simulink model "MotMappedP1"  (R2020a)
settings: Solver=VariableStepAuto  StartTime=0.0  StopTime=inf  RelTol=1e-3  EnableMultiTasking=on
model workspace (MAT data in the model file):
  T_eff_bp = [0 20 40 60 80 100 120 140 160 180 200]
  T_t = [200 200 200 200 190.9859317 143.2394488 114.591559 95.49296586 81.85111359 71.61972439 63.66197724 57.29577951 52.08707228 47.74648293]
  Tc = 0.02
  efficiency_table = [52  78  80  82  82  80  78  78  76  74  70; 52  78  80  82  82  80  78  78  76  74  70; 52  78  84  86  86  86  86  84  84  82  82; 52  80  86  86  88  88  88  86  86  84  84; 52  80  86  88  88  88  88  88  86  86  86; 52  80  86  88  90  90  90  90  88  88  88; 52  82  88  90  91  91  92  92  92  91  91; 52  82  88  91  91  92  93  93  93  93  93; 52  84  90  92  92  93  93  93  93  93  93; 62  86  91  93  93  93  93  93  93  93  93; 66  86  91  93  93  93  93  93  93  93  93; 70  86  92  93  93  93  93  93  93  93  93; 70  86  92  93  93  93  93  93  93  93  93; 72  86  91  93  93  93  93  93  93  93  93]
  power_max = 30000
  torque_max = 200
  w_eff_bp = [0 500 1000 1432.391138 1500 2000 2500 3000 3500 4000 4500 5000 5500 6000]
libraries: autolibmappedmotor x1
settings Model: ModifiedByFormat=The MathWorks, Inc.  PauseTimes=10  Creator=The MathWorks, Inc.  LastModifiedBy=The MathWorks, Inc.
settings SolverCC: AutoInsertRateTranBlk=on  DecoupledContinuousIntegration=on
settings DataIOCC: DSMLogging=off  ReturnWorkspaceOutputs=off
settings DebuggingCC: ArithmeticOperatorsInVariantConditions=warning
settings ModelReferenceCC: PropagateSignalLabelsOutOfModel=off
settings SFSimCC: SimUseLocalCustomCode=off  CustomCodeUndefinedFunction=UseInterfaceOnly
settings RTWCC: RTWUseLocalCustomCode=off
settings CodeAppCC: StateflowObjectComments=on
settings GRTTargetCC: TargetLangStandard=C89/C90 (ANSI)
settings ConfigComp: CovMetricSettings=dsw  CovHtmlReporting=on  CovSaveCumulativeToWorkspaceVar=on  CovSaveSingleToWorkspaceVar=on  CovShowResultsExplorer=off  CovExternalEMLEnable=off
settings SimscapeCC: SimscapeNormalizeSystem=off

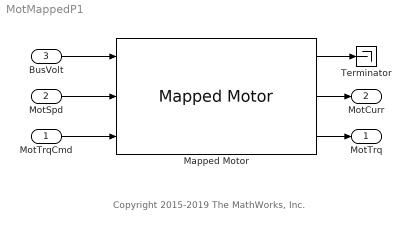
== system MotMappedP1 ==
  note: Copyright 2015-2019 The MathWorks, Inc.
  MotTrqCmd : Inport
  MotSpd : Inport  Port=2
  BusVolt : Inport  Port=3
  Mapped Motor : autolibmappedmotor/Mapped Motor  port_config=Speed  param_by=Tabulated torque-speed envelope  w_t=w_eff_bp.*pi/30  T_t=T_t  torque_max=torque_max  power_max=power_max  Tc=Tc  param_loss=Tabulated efficiency data  eff=100  w_eff=375  T_eff=0.08  Piron=0  Pbase=0  w_eff_bp=w_eff_bp.*pi/30  T_eff_bp=T_eff_bp  Temp_eff_bp=[233.15 293.15 373.15]  losses_table=[1 2;3 4]  losses_table_3d=cat(3,1.05*[1.49 1.67 2.21 3.10; 0.42 0.69 1.14 2.03; 0.06 0.24 0.78 1.68; 0.42 0.69 1.14 2.03; 1.49 1.67 2.21 3.10],[1.49 1.67 2.21 3.10; 0.42 0.69 1.14 2.03; 0.06 0.24 0.78 1.68; 0.42 0.69 1.14 2.03; 1.49 1.67 2.21 3.10],1.03*[1.49 1.67 2.21 3.10; 0.42 0.69 1.14 2.03; 0.06 0.24 0.78 1.68; 0.42 0.69 1.14 2.03; 1.49 1.67 2.21 3.10])  efficiency_table=efficiency_table  efficiency_table_3d=cat(3,90*ones(5,4),95*ones(5,4),92*ones(5,4))  J=5e-6  b=1e-5  omega_o=0  T_t_extended=[47.74648293 52.08707228 57.29577951 63.66197724 71.61972439 81.85111359 95.49296586 114.591559 143.2394488 190.9859317 200 200 200 200 200 200 200 190.9859317 143.2394488 114.591559 95.49296586 81.85111359 71.61972439 63.66197724 57.29577951 52.08707228 47.74648293]  w_t_extended=[-628.318530717959 -575.958653158129 -523.598775598299 -471.238898038469 -418.879020478639 -366.519142918809 -314.159265358979 -261.799387799149 -209.43951023932 -157.07963267949 -149.999649206931 -104.71975511966 -52.3598775598299 0 52.3598775598299 104.71975511966 149.999649206931 157.07963267949 209.43951023932 261.799387799149 314.159265358979 366.519142918809 418.879020478639 471.238898038469 523.598775598299 575.958653158129 628.318530717959]  KLossIron=0  KLossCopper=0  x_w_eff_vec=[-628.318530717959 -575.958653158129 -523.598775598299 -471.238898038469 -418.879020478639 -366.519142918809 -314.159265358979 -261.799387799149 -209.43951023932 -157.07963267949 -149.999649206931 -104.71975511966 -52.3598775598299 0 52.3598775598299 104.71975511966 149.999649206931 157.07963267949 209.43951023932 261.799387799149 314.159265358979 366.519142918809 418.879020478639 471.238898038469 523.598775598299 575.958653158129 628.318530717959]  x_T_eff_vec=[-200 -180 -160 -140 -120 -100 -80 -60 -40 -20 0 20 40 60 80 100 120 140 160 180 200]  x_tmp_eff_vec=[233.15 293.15 373.15]  x_losses_mat=[9458.558526937 8512.7026742433 7566.8468215496 6620.9909688559 5675.1351161622 4729.2792634685 3783.4234107748 2837.5675580811 2485.6557259172 2045.68823954684 0 1759.29188601028 2261.94671058465 2638.93782901542 3518.58377202057 4398.22971502571 5277.87565803085 6157.52160103599 7037.16754404113 7916.81348704627 8796.45943005141;8670.34531635892 7803.31078472303 6936.27625308713 6069.24172145124 5202.20718981535 4335.17265817946 3468.13812654357 2601.10359490768 2003.3344457674 1875.21421958461 0 1612.68422884276 1843.06769010601 2419.02634326414 3225.36845768552 4031.7105721069 4838.05268652828 5644.39480094966 6450.73691537104 7257.07902979242 8063.4211442138;7882.13210578084 7093.91889520275 6305.70568462467 5517.49247404659 4729.2792634685 3941.06605289042 3152.85284231233 2364.63963173425 1821.21313251582 1704.74019962237 0 1466.07657167524 1675.51608191456 2199.11485751285 2932.15314335047 3665.19142918809 4398.22971502571 5131.26800086333 5864.30628670094 6597.34457253856 7330.38285837618;7093.91889520275 6384.52700568248 5675.1351161622 4965.74322664193 4256.35133712165 3546.95944760138 2837.5675580811 2128.17566856083 1864.2417944379 1534.26617966013 0 1319.46891450771 1696.46003293849 1979.20337176157 2638.93782901542 3298.67228626928 3958.40674352314 4618.14120077699 5277.87565803085 5937.61011528471 6597.34457253856;6305.70568462467 5675.1351161622 5044.56454769974 4413.99397923727 3783.4234107748 3152.85284231233 2522.28227384987 1891.7117053874 1657.10381727813 1363.7921596979 0 1172.86125734019 1507.9644737231 1759.29188601028 2345.72251468038 2932.15314335047 3518.58377202057 4105.01440069066 4691.44502936075 5277.87565803085 5864.30628670094;5517.49247404658 4965.74322664193 4413.99397923727 3862.24473183261 3310.49548442795 2758.74623702329 2549.69838552215 1912.27378914161 1628.97396852804 1396.26340159546 0 1172.86125734019 1466.07657167524 1759.29188601028 2345.72251468038 2565.63400043166 3078.76080051799 3591.88760060433 4105.01440069066 4618.14120077699 5131.26800086332;4729.2792634685 4256.35133712165 3783.4234107748 3310.49548442795 2837.5675580811 2731.81969877373 2485.6557259172 1864.2417944379 1713.59599286716 1379.23579913698 0 1130.97335529233 1507.9644737231 1696.46003293849 2261.94671058465 2513.27412287183 2638.93782901542 3078.760800518 3518.58377202057 3958.40674352314 4398.22971502571;5178.44942899416 4660.60448609474 3642.42626503164 3187.12298190269 2731.81969877373 2589.22471449708 2071.37977159766 1745.32925199433 1427.99666072263 1149.36316594749 0 942.477796076938 1256.63706143592 1570.7963267949 1884.95559215388 2356.19449019234 2513.27412287183 2932.15314335047 3351.03216382911 4241.15008234622 4712.38898038469;5711.98664289054 5140.78797860148 4569.58931431243 3257.94793705608 2792.52680319093 2327.10566932577 1861.68453546062 1713.59599286716 1363.7921596979 1047.1975511966 0 837.758040957278 1172.86125734019 1507.9644737231 1675.51608191456 2094.39510239319 2513.27412287183 2932.15314335047 4021.23859659494 4523.8934211693 5026.54824574367;5114.22059886711 4602.7985389804 4091.37647909369 2998.79298751753 2570.39398930074 2141.99499108395 1713.59599286716 1285.19699465037 1022.84411977342 785.398163397448 0 628.318530717959 879.645943005142 1130.97335529233 1507.9644737231 1884.95559215388 2261.94671058465 2638.93782901543 3518.58377202057 3958.40674352314 4398.22971502571;5714.27235074022 5142.8451156662 3906.96760725029 3418.596656344 2454.53971429523 2045.44976191269 1636.35980953016 1465.11285271886 976.741901812573 749.998246034654 0 599.998596827723 839.998035558812 1259.99705333822 1439.99663238654 1799.99579048317 2159.9949485798 2939.99312445584 3359.99214223525 4319.98989715961 4799.98877462179;4597.45266378994 4137.70739741095 3191.45920364677 2792.52680319093 2045.68823954684 1704.74019962237 1363.7921596979 1022.84411977342 797.864800911693 590.726823751927 0 460.766922526503 670.206432765823 879.645943005142 1172.86125734019 1466.07657167524 1759.29188601028 ...(+4852 chars)]  x_losses_mat_3d=cat(3,[3.255 2.3205 1.7535 1.5645 1.7535 2.3205 3.255;2.1315 1.197 0.7245 0.441 0.7245 1.197 2.1315;1.764 0.819 0.252 0.063 0.252 0.819 1.764;2.1315 1.197 0.7245 0.441 0.7245 1.197 2.1315;3.255 2.3205 1.7535 1.5645 1.7535 2.3205 3.255],[3.1 2.21 1.67 1.49 1.67 2.21 3.1;2.03 1.14 0.69 0.42 0.69 1.14 2.03;1.68 0.78 0.24 0.06 0.24 0.78 1.68;2.03 1.14 0.69 0.42 0.69 1.14 2.03;3.1 2.21 1.67 1.49 1.67 2.21 3.1],[3.193 2.2763 1.7201 1.5347 1.7201 2.2763 3.193;2.0909 1.1742 0.7107 0.4326 0.7107 1.1742 2.0909;1.7304 0.8034 0.2472 0.0618 0.2472 0.8034 1.7304;2.0909 1.1742 0.7107 0.4326 0.7107 1.1742 2.0909;3.193 2.2763 1.7201 1.5347 1.7201 2.2763 3.193])  CalLossMapData={}  CalLossWithTempMapData={}  aMode=aMode  RefBlkName='autolibmappedmotor/Mapped Motor'
      settings: SourceProductBaseCode=PW,MT,VE,VP
  Terminator : Terminator
  MotTrq : Outport  VectorParamsAs1DForOutWhenUnconnected=off
  MotCurr : Outport  Port=2  VectorParamsAs1DForOutWhenUnconnected=off
  wires:
  MotTrqCmd/1 -> Mapped Motor/3
  BusVolt/1 -> Mapped Motor/1
  MotSpd/1 -> Mapped Motor/2
  Mapped Motor/3 -> MotTrq/1
  Mapped Motor/2 -> MotCurr/1
  Mapped Motor/1 -> Terminator/1
